simulink model "vipabandonedobj"  (R2015b)
settings: Solver=FixedStepDiscrete  StartTime=0.0  StopTime=inf  RelTol=1e-3
model workspace (MATLAB code in the model file):
  | maxNumObj = 200;  % maximum number of objects to track
values from neighbouring files (symbols this model uses):
  roi = roi( aspectRatio > 0.25 & aspectRatio < 1 ,:)    [OCRExample.m]    (also in videopattern_gettemplate.m = api.getPosition())
undefined symbols (not defined in the file or in its folder): gray, Rec, SDTV, strel
libraries: visiontextngfix x6, visionsinks x3, visionconversions x2, visionstatistics x1, simulink x1, visionmorphops x1, dspvision x1, vipmisc x1
CloseFcn:
  | clear line_row;
settings Model: FPTRunName=Active  ExtModeAutoUpdateStatusClock=off  Creator=The MathWorks, Inc.  LastModifiedBy=The MathWorks, Inc.
settings DataIOCC: LimitDataPoints=off  SaveFormat=Array  SaveOutput=off  SignalLogging=off  SaveTime=off  SignalLoggingName=sigsOut
settings OptimizationCC: ExpressionDepthLimit=2147483647  InitFltsAndDblsToZero=on  EfficientMapNaN2IntZero=off  BufferReusableBoundary=off
settings DebuggingCC: AlgebraicLoopMsg=none  SaveWithParameterizedLinksMsg=none  CheckExecutionContextPreStartOutputMsg=on  CheckExecutionContextRuntimeOutputMsg=on  SignalResolutionControl=TryResolveAllWithWarning  InheritedTsInSrcMsg=none  MultiTaskDSMMsg=warning  MultiTaskCondExecSysMsg=none  ParameterPrecisionLossMsg=none  FcnCallInpInsideContextMsg=UseLocalSettings  BusObjectLabelMismatch=none  StateNameClashWarn=warning
settings HardwareCC: ProdBitPerPointer=32  ProdLargestAtomicFloat=None  ProdIntDivRoundTo=Undefined  ProdEndianess=Unspecified  ProdWordSize=32  ProdHWDeviceType=32-bit Generic  TargetBitPerLong=64  TargetBitPerPointer=64  TargetLongLongMode=on  TargetIntDivRoundTo=Zero  TargetEndianess=LittleEndian  TargetWordSize=64  TargetHWDeviceType=Generic->MATLAB Host Computer  ProdEqTarget=off
settings SFSimCC: SimParseCustomCode=off
settings GRTTargetCC: TargetFcnLib=ansi_tfl_tmw.mat  GeneratePreprocessorConditionals=Disable all  CombineOutputUpdateFcns=off  GRTInterface=on
settings ConfigComp: CovModelRefEnable=Off

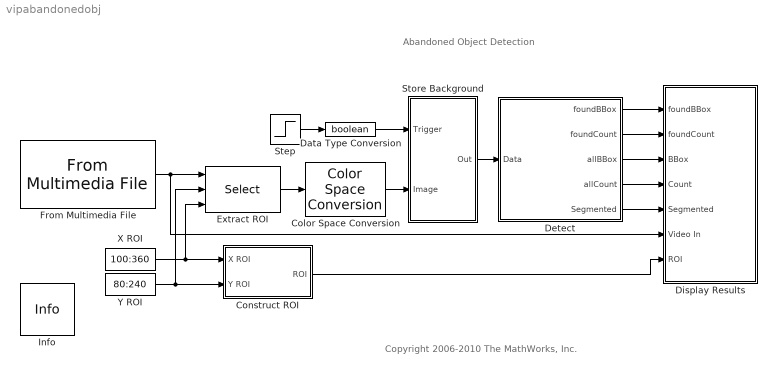
== system vipabandonedobj ==
  note: Abandoned Object Detection
  note: Copyright 2006-2010 The MathWorks, Inc.
  Color Space Conversion : visionconversions/Color Space  Conversion  conversion=Obsolete  conversionActive=R'G'B' to Y'CbCr  wp_str=D65  rec=Rec. 601 (SDTV)  sys=1125/60/2:1  imagePorts=One multidimensional signal
  Construct ROI : Subsystem
  Data Type Conversion : DataTypeConversion  OutDataTypeStr=boolean
  Detect : Subsystem  TreatAsAtomicUnit=on
      settings: RTWMemSecFuncInitTerm=Default  RTWMemSecFuncExecute=Default  RTWMemSecDataConstants=Default  RTWMemSecDataInternal=Default  RTWMemSecDataParameters=Default
  Display Results : Subsystem
      settings: RTWMemSecFuncInitTerm=Default  RTWMemSecFuncExecute=Default  RTWMemSecDataConstants=Default  RTWMemSecDataInternal=Default  RTWMemSecDataParameters=Default
  Extract ROI : Selector  NumberOfDimensions=3  IndexOptions=Index vector (port),Index vector (port),Select all  Indices=[roi(1):roi(3)],[roi(2):roi(4)],[]  OutputSizes=1
  From Multimedia File : dspvision/From Multimedia File  inputFilename=viptrain.avi  loop=on  numPlays=inf  outputStreams=Video only  videoDataType=single  audioDataType=int16  inheritSampleTime=on  userDefinedSampleTime=1/30  noAudioOutput=off  isIntensityVideo=off  fourcc=RGB  colorVideoFormat=One multidimensional signal  outputEOF=off  dataOrg=Column-major  audioFrameSize=1024  computeAudioFrameSize=off  outSamplingMode=Frame based
  Info : vipmisc/Info  SystemSampleTime=-1
  Step : Step  Time=eps
  Store Background : Subsystem
  X ROI : Constant  Value=100:360
  Y ROI : Constant  Value=80:240
  wires:
  From Multimedia File/1 -> Extract ROI/1, Display Results/6(Video In)
  Data Type Conversion/1 -> Store Background/1(Trigger)
  Detect/5(Segmented) -> Display Results/5(Segmented)
  Detect/4(allCount) -> Display Results/4(Count)
  Detect/3(allBBox) -> Display Results/3(BBox)
  Detect/1(foundBBox) -> Display Results/1(foundBBox)
  Detect/2(foundCount) -> Display Results/2(foundCount)
  Store Background/1(Out) -> Detect/1(Data)
  Extract ROI/1 -> Color Space Conversion/1
  Color Space Conversion/1 -> Store Background/2(Image)
  X ROI/1 -> Construct ROI/1("X ROI "), Extract ROI/3
  Y ROI/1 -> Construct ROI/2(Y ROI), Extract ROI/2
  Construct ROI/1(ROI) -> Display Results/7(ROI)
  Step/1 -> Data Type Conversion/1

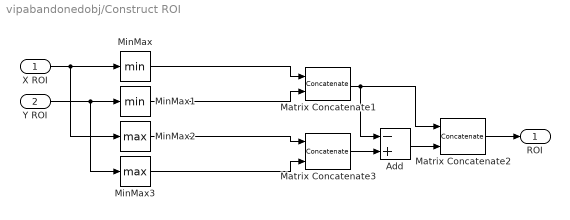
== system vipabandonedobj/Construct ROI ==
  "X ROI " : Inport
  Y ROI : Inport  Port=2
  Add : Sum  Inputs=-+
  Matrix Concatenate1 : Concatenate  Mode=Multidimensional array  ConcatenateDimension=2
  Matrix Concatenate2 : Concatenate  Mode=Multidimensional array  ConcatenateDimension=2
  Matrix Concatenate3 : Concatenate  Mode=Multidimensional array  ConcatenateDimension=2
  MinMax : MinMax
  MinMax1 : MinMax
  MinMax2 : MinMax  Function=max
  MinMax3 : MinMax  Function=max
  ROI : Outport
  wires:
  "X ROI "/1 -> MinMax/1, MinMax2/1
  MinMax/1 -> Matrix Concatenate1/1
  MinMax1/1 -> Matrix Concatenate1/2
  Matrix Concatenate1/1 -> Add/1, Matrix Concatenate2/1
  Matrix Concatenate2/1 -> ROI/1
  Y ROI/1 -> MinMax1/1, MinMax3/1
  MinMax2/1 -> Matrix Concatenate3/1
  MinMax3/1 -> Matrix Concatenate3/2
  Matrix Concatenate3/1 -> Add/2
  Add/1 -> Matrix Concatenate2/2

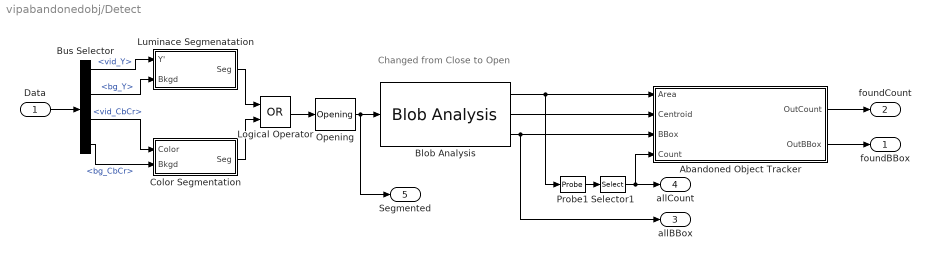
== system vipabandonedobj/Detect ==
  note: Changed from Close to Open
  Data : Inport
  Abandoned Object Tracker : Subsystem  mask(Abandoned Object Tracker){alarmCount=45, maxConsecutiveMiss=4, areaChangeFraction=15-2, centroidChangeFraction=20-2, minPersistenceRatio=0.7, maxNumObj=maxNumObj}
      mask prompts: alarmCount "Number of frames that an object remains stationary before alarm is raised:"; maxConsecutiveMiss "Maximum consecutive misses tolerance in number of frames:"; areaChangeFraction "Area change tolerance in %:"; centroidChangeFraction "Centroid change tolerance in %:"; minPersistenceRatio "Minimum persistence ratio:"; maxNumObj "Maximum number of objectes:"
      mask help: Detects objects that remain stationary for a specified period of time. This is accomplished through tracking area, centroid and bounding box of each object.
      mask Help: This block illustrates use of EML for multiple object tracking.  Look under its mask to see the implementation details.
      mask Display: disp('Abandoned Object\nTracker');
  Blob Analysis : visionstatistics/Blob Analysis  Tag=vipblks_row_conv  area=on  centroid=on  bBox=on  majorAxis=off  minorAxis=off  angle=off  eccentricity=off  equivDiameterSq=off  extent=off  perimeter=off  maxBlobs=maxNumObj  warnIfNumBlobsExceeded=on  isCount=off  useMinArea=on  minArea=100  useMaxArea=on  maxArea=2500  excludeBorderBlob=on  outDT=double  isOutVarDim=on  isFill=on  fillValues=-1  conn=8  isLabel=off  outputMode=Binary point scaling  outputWordLength=32  outputFracLength=16  firstCoeffMode=Binary point scaling  firstCoeffWordLength=16  firstCoeffFracLength=14  secondCoeffMode=Binary point scaling  secondCoeffWordLength=32  secondCoeffFracLength=16  accumMode=Binary point scaling  accumWordLength=32  accumFracLength=0  prodOutputMode=Binary point scaling  prodOutputWordLength=32  prodOutputFracLength=16  roundingMode=Floor  overflowMode=off
  Bus Selector : BusSelector  OutputSignals=vid_Y,bg_Y,vid_CbCr,bg_CbCr
  Color Segmentation : Subsystem
      settings: RTWMemSecFuncInitTerm=Default  RTWMemSecFuncExecute=Default  RTWMemSecDataConstants=Default  RTWMemSecDataInternal=Default  RTWMemSecDataParameters=Default
  Logical Operator : Logic  Operator=OR  AllPortsSameDT=off  OutDataTypeStr=boolean
  Luminace Segmenatation : Subsystem
      settings: RTWMemSecFuncInitTerm=Default  RTWMemSecFuncExecute=Default  RTWMemSecDataConstants=Default  RTWMemSecDataInternal=Default  RTWMemSecDataParameters=Default
  Opening : visionmorphops/Opening  nhoodsrc=Specify via dialog  strel=strel('square',3)
  Probe1 : Probe  ProbeWidth=off  ProbeSampleTime=off  ProbeComplexSignal=off  ProbeSignalDimensions=on  ProbeDimensionsDataType=int32
  Selector1 : Selector  InputPortWidth=2  IndexOptions=Index vector (dialog)  Indices=1  OutputSizes=1
  foundBBox : Outport
  foundCount : Outport  Port=2
  allBBox : Outport  Port=3
  allCount : Outport  Port=4
  Segmented : Outport  Port=5
  wires:
  Abandoned Object Tracker/1(OutCount) -> foundCount/1
  Abandoned Object Tracker/2(OutBBox) -> foundBBox/1
  Data/1 -> Bus Selector/1
  Bus Selector/1 -> Luminace Segmenatation/1(Y')  "<vid_Y>"
  Bus Selector/2 -> Luminace Segmenatation/2(Bkgd)  "<bg_Y>"
  Bus Selector/3 -> Color Segmentation/1(Color)  "<vid_CbCr>"
  Bus Selector/4 -> Color Segmentation/2(Bkgd)  "<bg_CbCr>"
  Luminace Segmenatation/1(Seg) -> Logical Operator/1
  Color Segmentation/1(Seg) -> Logical Operator/2
  Blob Analysis/1 -> Abandoned Object Tracker/1(Area), Probe1/1
  Blob Analysis/2 -> Abandoned Object Tracker/2(Centroid)
  Blob Analysis/3 -> Abandoned Object Tracker/3(BBox), allBBox/1
  Logical Operator/1 -> Opening/1
  Opening/1 -> Segmented/1, Blob Analysis/1
  Selector1/1 -> allCount/1, Abandoned Object Tracker/4(Count)
  Probe1/1 -> Selector1/1

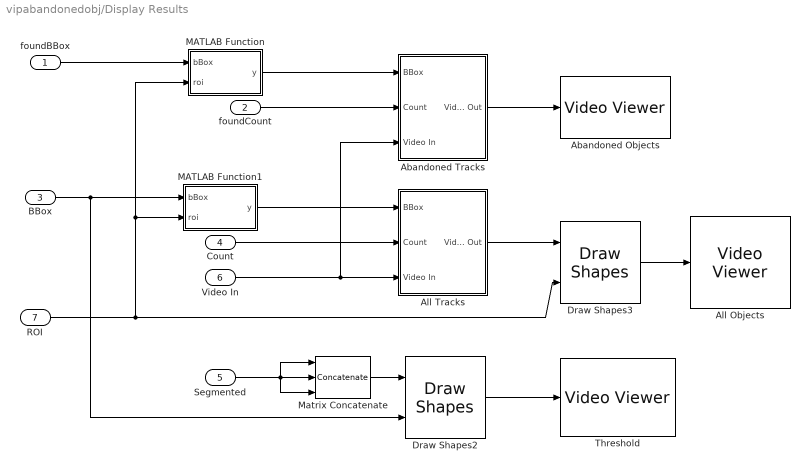
== system vipabandonedobj/Display Results ==
  foundBBox : Inport
  foundCount : Inport  Port=2
  BBox : Inport  Port=3
  Count : Inport  Port=4
  Segmented : Inport  Port=5
  Video In : Inport  Port=6
  ROI : Inport  Port=7
  Abandoned Objects : visionsinks/Video Viewer  inputType=Obsolete7b  imagePorts=One multidimensional signal  useColorMap=off  colormapValue=gray(256)  specRange=off  minInputVal=0  maxInputVal=255  FigPos=[629 387 362 261]  AxisZoom=on  trueSizedOnce=on  OpenAtMdlStart=on  DefaultConfigurationName=vipscopes.VideoViewerScopeCfg
  Abandoned Tracks : Subsystem
      settings: RTWMemSecFuncInitTerm=Default  RTWMemSecFuncExecute=Default  RTWMemSecDataConstants=Default  RTWMemSecDataInternal=Default  RTWMemSecDataParameters=Default
  All Objects : visionsinks/Video Viewer  inputType=Obsolete7b  imagePorts=One multidimensional signal  useColorMap=off  colormapValue=gray(256)  specRange=off  minInputVal=0  maxInputVal=255  FigPos=[75 390 360 261]  AxisZoom=on  trueSizedOnce=on  OpenAtMdlStart=on  DefaultConfigurationName=vipscopes.VideoViewerScopeCfg
  All Tracks : Subsystem
      settings: RTWMemSecFuncInitTerm=Default  RTWMemSecFuncExecute=Default  RTWMemSecDataConstants=Default  RTWMemSecDataInternal=Default  RTWMemSecDataParameters=Default
  Draw Shapes2 : visiontextngfix/Draw Shapes  shape=Rectangles  fill=off  lineWidth=1  fillClrSource=Specify via dialog  display=User-specified value  intensity=200  color=[0 1 0]  opacity=0.5  viewport=Entire image  antialiasing=off  inType=Obsolete  imagePorts=One multidimensional signal  prodOutputMode=Binary point scaling  prodOutputWordLength=32  prodOutputFracLength=14  memoryMode=Specify word length  memoryWordLength=16  memoryFracLength=14  roundingMode=Floor  overflowMode=off
  Draw Shapes3 : visiontextngfix/Draw Shapes  shape=Rectangles  fill=off  lineWidth=1  fillClrSource=Specify via dialog  display=User-specified value  intensity=200  color=[1 1 0]  opacity=0.5  viewport=Entire image  antialiasing=off  inType=Obsolete  imagePorts=One multidimensional signal  prodOutputMode=Binary point scaling  prodOutputWordLength=32  prodOutputFracLength=14  memoryMode=Specify word length  memoryWordLength=16  memoryFracLength=14  roundingMode=Floor  overflowMode=off
  MATLAB Function : MATLAB Function  TreatAsAtomicUnit=on
  MATLAB Function1 : MATLAB Function  TreatAsAtomicUnit=on
  Matrix Concatenate : Concatenate  NumInputs=3  Mode=Multidimensional array  ConcatenateDimension=3
  Threshold : visionsinks/Video Viewer  inputType=Obsolete7b  imagePorts=One multidimensional signal  useColorMap=off  colormapValue=gray(256)  specRange=off  minInputVal=0  maxInputVal=255  FigPos=[72 704 261 183]  AxisZoom=on  trueSizedOnce=on  OpenAtMdlStart=on  DefaultConfigurationName=vipscopes.VideoViewerScopeCfg
  wires:
  Draw Shapes2/1 -> Threshold/1
  Matrix Concatenate/1 -> Draw Shapes2/1
  Segmented/1 -> Matrix Concatenate/3, Matrix Concatenate/2, Matrix Concatenate/1
  Draw Shapes3/1 -> All Objects/1
  All Tracks/1(Video Out) -> Draw Shapes3/1
  Abandoned Tracks/1(Video Out) -> Abandoned Objects/1
  ROI/1 -> MATLAB Function/2(roi), MATLAB Function1/2(roi), Draw Shapes3/2
  foundCount/1 -> Abandoned Tracks/2(Count)
  Video In/1 -> Abandoned Tracks/3(Video In), All Tracks/3(Video In)
  Count/1 -> All Tracks/2(Count)
  BBox/1 -> MATLAB Function1/1(bBox), Draw Shapes2/2
  MATLAB Function1/1(y) -> All Tracks/1(BBox)
  MATLAB Function/1(y) -> Abandoned Tracks/1(BBox)
  foundBBox/1 -> MATLAB Function/1(bBox)

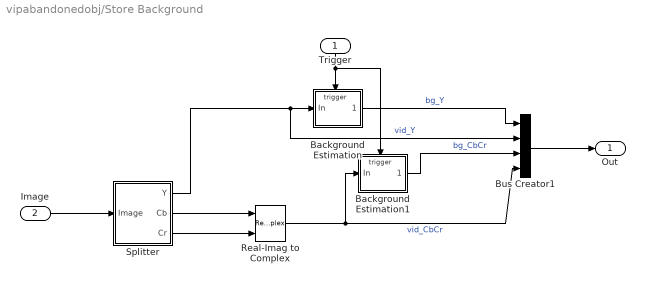
== system vipabandonedobj/Store Background ==
  Trigger : Inport
  Image : Inport  Port=2
  Background Estimation : Subsystem  TreatAsAtomicUnit=on  mask{initCond=0}
      mask prompts: initCond "Initial Condition"
  Background Estimation1 : Subsystem  TreatAsAtomicUnit=on  mask{initCond=0}
      mask prompts: initCond "Initial Condition"
  Bus Creator1 : BusCreator  Inputs=4
  Real-Imag to Complex : RealImagToComplex
  Splitter : Subsystem
  Out : Outport
  wires:
  Image/1 -> Splitter/1(Image)
  Splitter/3(Cr) -> Real-Imag to Complex/2
  Splitter/2(Cb) -> Real-Imag to Complex/1
  Bus Creator1/1 -> Out/1
  Trigger/1 -> Background Estimation/Trigger, Background Estimation1/Trigger
  Background Estimation1/1(" ") -> Bus Creator1/3  "bg_CbCr"
  Background Estimation/1(" ") -> Bus Creator1/1  "bg_Y"
  Real-Imag to Complex/1 -> Bus Creator1/4, Background Estimation1/1(In)  "vid_CbCr"
  Splitter/1(Y) -> Bus Creator1/2, Background Estimation/1(In)  "vid_Y"

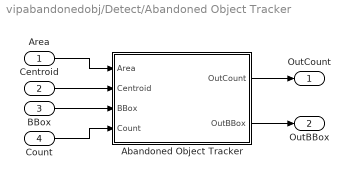
== system vipabandonedobj/Detect/Abandoned Object Tracker ==
  Area : Inport
  Centroid : Inport  Port=2
  BBox : Inport  Port=3
  Count : Inport  Port=4
  Abandoned Object Tracker : MATLAB Function  TreatAsAtomicUnit=on
  OutCount : Outport
  OutBBox : Outport  Port=2
  wires:
  Centroid/1 -> Abandoned Object Tracker/2(Centroid)
  BBox/1 -> Abandoned Object Tracker/3(BBox)
  Abandoned Object Tracker/1(OutCount) -> OutCount/1
  Abandoned Object Tracker/2(OutBBox) -> OutBBox/1
  Area/1 -> Abandoned Object Tracker/1(Area)
  Count/1 -> Abandoned Object Tracker/4(Count)

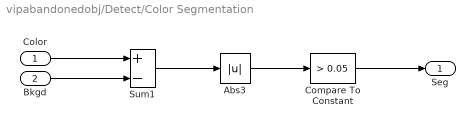
== system vipabandonedobj/Detect/Color Segmentation ==
  Color : Inport
  Bkgd : Inport  Port=2
  Abs3 : Abs  SaturateOnIntegerOverflow=on
  Compare To Constant : simulink/Logic and Bit Operations/Compare To Constant  relop=>  const=0.05  OutDataTypeStr=boolean  ZeroCross=off
  Sum1 : Sum  Inputs=+-  SaturateOnIntegerOverflow=on  InputSameDT=on  OutDataTypeStr=Inherit: Same as first input
  Seg : Outport
  wires:
  Bkgd/1 -> Sum1/2
  Color/1 -> Sum1/1
  Sum1/1 -> Abs3/1
  Compare To Constant/1 -> Seg/1
  Abs3/1 -> Compare To Constant/1

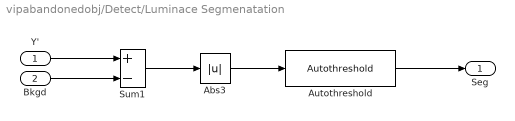
== system vipabandonedobj/Detect/Luminace Segmenatation ==
  Y' : Inport
  Bkgd : Inport  Port=2
  Abs3 : Abs  SaturateOnIntegerOverflow=on
  Autothreshold : visionconversions/Autothreshold  operator=>  threshOut=off  effMetricOut=off  userDefinedRange=off  umin=0  umax=100  outOfRngOpt=Warn and saturate  scaleThreshold=on  scaleFactor=1.3  P1Mode=Specify word length  P1WordLength=32  P1FracLength=30  P2Mode=Specify word length  P2WordLength=32  P2FracLength=22  P3Mode=Specify word length  P3WordLength=32  P3FracLength=14  P4Mode=Binary point scaling  P4WordLength=32  P4FracLength=15  Q1Mode=Specify word length  Q1WordLength=32  Q1FracLength=16  EMMode=Specify word length  EMWordLength=16  EMFracLength=14  roundingMode=Floor  overflowMode=off
  Sum1 : Sum  Inputs=+-  SaturateOnIntegerOverflow=on  InputSameDT=on  OutDataTypeStr=Inherit: Same as first input
  Seg : Outport
  wires:
  Abs3/1 -> Autothreshold/1
  Autothreshold/1 -> Seg/1
  Sum1/1 -> Abs3/1
  Y'/1 -> Sum1/1
  Bkgd/1 -> Sum1/2

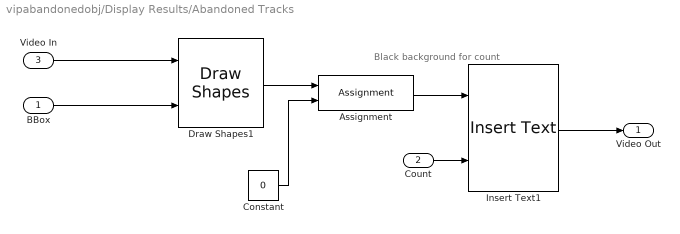
== system vipabandonedobj/Display Results/Abandoned Tracks ==
  note: Black background
      | for count
  BBox : Inport
  Count : Inport  Port=2
  Video In : Inport  Port=3
  Assignment : Assignment  NumberOfDimensions=3  IndexOptions=Index vector (dialog),Index vector (dialog),Assign all  Indices=[1:15],[1:30],[]  OutputSizes=1, 1
  Constant : Constant  Value=0  VectorParams1D=off  OutDataTypeStr=Inherit: Inherit via back propagation
  Draw Shapes1 : visiontextngfix/Draw Shapes  shape=Rectangles  fill=on  lineWidth=1  fillClrSource=Specify via dialog  display=User-specified value  intensity=200  color=[1 0 0]  opacity=0.5  viewport=Entire image  antialiasing=off  inType=Obsolete  imagePorts=One multidimensional signal  prodOutputMode=Binary point scaling  prodOutputWordLength=32  prodOutputFracLength=14  memoryMode=Specify word length  memoryWordLength=16  memoryFracLength=14  roundingMode=Floor  overflowMode=off
  Insert Text1 : visiontextngfix/Insert Text  inputType=Obsolete  theText='%4d'  getTextLocFrom=Specify via dialog  textLoc=[0 0]  getTextColorFrom=Specify via dialog  textColor=[1 1 1]  getTextIntensityFrom=Specify via dialog  textIntensity=0  getTextOpacityFrom=Specify via dialog  textOpacity=1.0  dummyVar2=0  dummyVar3=0  dummyVar4=0  imagePorts=One multidimensional signal  isInputTransposed=off  fontFace=LucidaSansRegular  dummyVar1=0  blockFontSize=12  antiAliased=on
  Video Out : Outport
  wires:
  Constant/1 -> Assignment/2
  Insert Text1/1 -> Video Out/1
  Video In/1 -> Draw Shapes1/1
  Assignment/1 -> Insert Text1/1
  Draw Shapes1/1 -> Assignment/1
  BBox/1 -> Draw Shapes1/2
  Count/1 -> Insert Text1/2

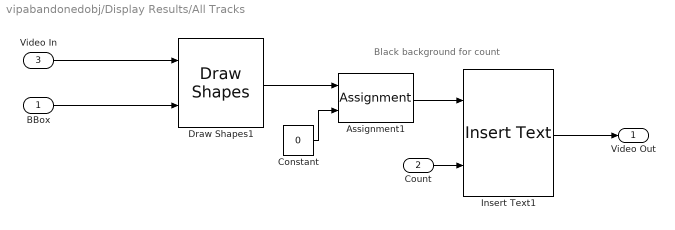
== system vipabandonedobj/Display Results/All Tracks ==
  note: Black background
      | for count
  BBox : Inport
  Count : Inport  Port=2
  Video In : Inport  Port=3
  Assignment1 : Assignment  NumberOfDimensions=3  IndexOptions=Index vector (dialog),Index vector (dialog),Assign all  Indices=[1:15],[1:30],[]  OutputSizes=1, 1
  Constant : Constant  Value=0  VectorParams1D=off  OutDataTypeStr=Inherit: Inherit via back propagation
  Draw Shapes1 : visiontextngfix/Draw Shapes  shape=Rectangles  fill=off  lineWidth=1  fillClrSource=Specify via dialog  display=User-specified value  intensity=200  color=[0 1 0]  opacity=0.5  viewport=Entire image  antialiasing=off  inType=Obsolete  imagePorts=One multidimensional signal  prodOutputMode=Binary point scaling  prodOutputWordLength=32  prodOutputFracLength=14  memoryMode=Specify word length  memoryWordLength=16  memoryFracLength=14  roundingMode=Floor  overflowMode=off
  Insert Text1 : visiontextngfix/Insert Text  inputType=Obsolete  theText='%4d'  getTextLocFrom=Specify via dialog  textLoc=[0 0]  getTextColorFrom=Specify via dialog  textColor=[1 1 1]  getTextIntensityFrom=Specify via dialog  textIntensity=0  getTextOpacityFrom=Specify via dialog  textOpacity=1.0  dummyVar2=0  dummyVar3=0  dummyVar4=0  imagePorts=One multidimensional signal  isInputTransposed=off  fontFace=LucidaSansRegular  dummyVar1=0  blockFontSize=12  antiAliased=on
  Video Out : Outport
  wires:
  Constant/1 -> Assignment1/2
  Insert Text1/1 -> Video Out/1
  Count/1 -> Insert Text1/2
  Video In/1 -> Draw Shapes1/1
  BBox/1 -> Draw Shapes1/2
  Draw Shapes1/1 -> Assignment1/1
  Assignment1/1 -> Insert Text1/1

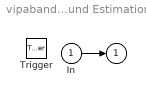
== system vipabandonedobj/Store Background/Background Estimation ==
  In : Inport
  Trigger : TriggerPort  ZeroCross=off
  " " : Outport  InitialOutput=initCond
  wires:
  In/1 -> " "/1

== system vipabandonedobj/Store Background/Background Estimation1 ==
  In : Inport
  Trigger : TriggerPort  ZeroCross=off
  " " : Outport  InitialOutput=initCond
  wires:
  In/1 -> " "/1

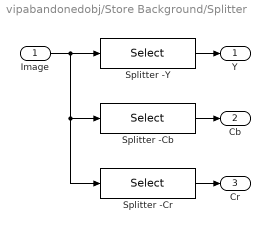
== system vipabandonedobj/Store Background/Splitter ==
  Image : Inport
  Splitter -Cb : Selector  NumberOfDimensions=3  IndexOptions=Select all,Select all,Index vector (dialog)  Indices=[],[],[2]  OutputSizes=1
  Splitter -Cr : Selector  NumberOfDimensions=3  IndexOptions=Select all,Select all,Index vector (dialog)  Indices=[],[],[3]  OutputSizes=1
  Splitter -Y : Selector  NumberOfDimensions=3  IndexOptions=Select all,Select all,Index vector (dialog)  Indices=[],[],[1]  OutputSizes=1
  Y : Outport
  Cb : Outport  Port=2
  Cr : Outport  Port=3
  wires:
  Image/1 -> Splitter -Cr/1, Splitter -Cb/1, Splitter -Y/1
  Splitter -Y/1 -> Y/1
  Splitter -Cb/1 -> Cb/1
  Splitter -Cr/1 -> Cr/1

== matlab function vipabandonedobj/Detect/Abandoned Object Tracker/Abandoned Object Tracker ==
  data: Area input; OutCount output; Centroid input; BBox input; Count input; OutBBox output size=size(BBox); areaChangeFraction parameter; centroidChangeFraction parameter; maxConsecutiveMiss parameter; minPersistenceRatio parameter; alarmCount parameter; maxNumObj parameter
%% This block implements an abandoned object tracker.
%%
%% Note:  Inputs that start with capital letter are represented as ports
%%        while inputs that start with lower case are mask parameters
%%

function [OutCount, OutBBox] = ObjTracker(Area, Centroid, BBox, Count, ...
    areaChangeFraction, centroidChangeFraction, maxConsecutiveMiss, ...
    minPersistenceRatio, alarmCount, maxNumObj)

% turn some inputs from percentages to fractions
areaChangeFraction = areaChangeFraction/100;
centroidChangeFraction = centroidChangeFraction/100;

% maximum number of objects is driven by output from Blob Analysis
maxNumTracks = length(Area);

% Initialize output variables
OutCount = zeros(1,class(Count));
OutBBox  = zeros(size(BBox),class(BBox));

% Declare integer valued, persistent elements of a Track
persistent track;
persistent idx_my;
if isempty(track)
    track = repmat(empty_track,maxNumObj, 1);
end
if isempty(idx_my)
    idx_my=1;
else
    idx_my = idx_my+1;
    if (idx_my==147)
        aaaa=1;
    end
end
%%%%%%%%%%%%%%%%%%%%%%%%%%% CORE ALGORITHM %%%%%%%%%%%%%%%%%%%%%%%%%%%%%

if (Count && ~isempty(BBox)) % if blobs were found
   % process tracks
   
   for i=1:double(Count) % scan through all the incoming blobs

       % quantize the values that we'll be tracking
       inCentroid = round(Centroid(i,1:2)/2);
       inArea     = round(double(Area(i))/2);
       
       found = false;
       for j=1:maxNumTracks
           T = track(j);
           if T.isTrackActive
               trackArea     = double(T.area);
               trackCentroid = double(T.centroid);
               
               areaRatio = abs(trackArea - inArea)/(trackArea+1);
               centDiff  = inCentroid - trackCentroid;
               centRatio = (centDiff*centDiff')/inArea;
                           
               % does this object belong to an existing track?
               if (areaRatio < areaChangeFraction) && ...
                  (centRatio < centroidChangeFraction)
                  found = true;
                  % update information about this object being tracked
                  track(j).justHit = true;
                  track(j).hitCount= track(j).hitCount + 1;
                  break;
               end
           end
       end
       
       if ~found % Then add to our list in first available position
           k = 1;
           for m=1:maxNumTracks
               if ~track(m).isTrackActive
                   k = m;
                   break;
               end
           end
           % fill track information
           track(k).area = int32(inArea);
           track(k).centroid = int32(inCentroid);
           track(k).bbox = int32(BBox(i,1:4));
           track(k).age = int32(1);
           track(k).hitCount = int32(1);
           track(k).missCount = int32(0);
           
           track(k).justHit = true;
           track(k).isTrackActive = true;
       end
   end
end

% Age existing tracks.  Update hit/miss counts and see which tracks were
% just hit.
for i=1:maxNumTracks
    if track(i).isTrackActive % Only process for active entries in list
        track(i).age = track(i).age + 1;
        % Find all tracks that were justHit and reset justHit flag
        % For the tracks that were just hit, increment hitCount and clear
        % missCount for the tracks that were not just hit, increment missCount
        if track(i).justHit
            track(i).justHit = false;
            track(i).missCount = int32(0); % clear consecutive misses
        else
            track(i).missCount = track(i).missCount + 1;
        end

        % Mark track for deletion if:
        %  * consecutive misses exceeds maxConsecutiveMiss
        %  * ratio of hitCount to age drops below minPersistenceRatio
        deleteMissFlag  = (track(i).missCount > maxConsecutiveMiss);
        deleteRatioFlag = (track(i).hitCount < track(i).age*...
            minPersistenceRatio);

        if (deleteMissFlag || deleteRatioFlag)
            track(i).isTrackActive = false;
        end
    end

    % Determine which objects are stationary
    if track(i).hitCount >= alarmCount
        OutCount = OutCount + 1;
        OutBBox(OutCount,:) = track(i).bbox;
    end
    if (OutCount ~=0)
        aaa=111;
    end
end
%------------------------------------------------------------------------%
function t = empty_track

t.area          = int32(0);
t.centroid      = int32([1 1]);
t.bbox          = int32([1 1 0 0]);
t.age           = int32(0);
t.hitCount      = int32(0);
t.missCount     = int32(0);
t.justHit       = false;
t.isTrackActive = false;

== matlab function vipabandonedobj/Display Results/MATLAB Function ==
  data: bBox input; y output size=size(bBox); roi input
function y = vAdd(bBox, roi)
%#codegen
% Add roi offset to the bounding boxes for display in the input image
y = bBox;
if (size(bBox,1)~=0)
    y(:,1) = bBox(:,1) + roi(1)-1;
    y(:,2) = bBox(:,2) + roi(2)-1;
end

== matlab function vipabandonedobj/Display Results/MATLAB Function1 ==
  data: bBox input; y output size=size(bBox); roi input
function y = vAdd(bBox, roi)
%#codegen
% Add roi offset to the bounding boxes for display in the input image
y = bBox;
if (size(bBox,1)~=0)
    y(:,1) = bBox(:,1) + roi(1)-1;
    y(:,2) = bBox(:,2) + roi(2)-1;
end
